simulink model "transfer_function"  (R2023a)
settings: Solver=VariableStepAuto  StartTime=0.0  StopTime=10.0  RelTol=1e-3
settings Model: Creator=HP  LastModifiedBy=HP

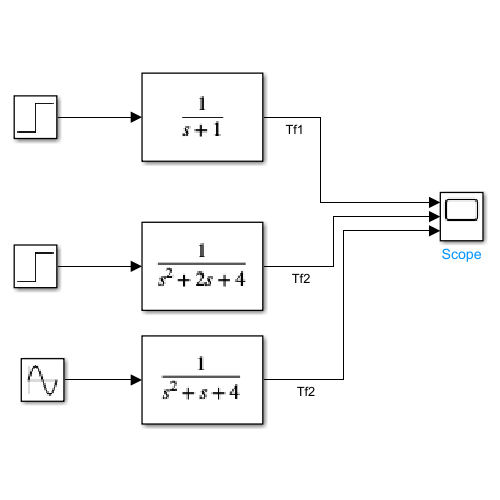
[thumbnail: Simulink's stored preview of the top-level diagram]
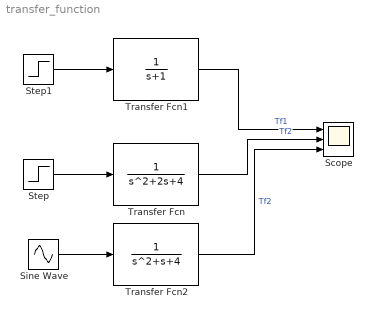
== system transfer_function ==
  Scope : Scope  NumInputPorts=3
  Sine Wave : Sin  SampleTime=0
  Step : Step  SampleTime=0
  Step1 : Step  SampleTime=0
  Transfer Fcn : TransferFcn  Denominator=[1 2 4]
  Transfer Fcn1 : TransferFcn  Denominator=[1 1]
  Transfer Fcn2 : TransferFcn  Denominator=[1 1 4]
  wires:
  Step/1 -> Transfer Fcn/1
  Transfer Fcn/1 -> Scope/2  "Tf2"
  Step1/1 -> Transfer Fcn1/1
  Transfer Fcn1/1 -> Scope/1  "Tf1"
  Transfer Fcn2/1 -> Scope/3  "Tf2"
  Sine Wave/1 -> Transfer Fcn2/1
